simulink model "ActingHealthCheck"  (R2023a)
settings: Solver=VariableStepAuto  StartTime=0.0  StopTime=10.0  RelTol=1e-3
settings Model: Creator=aan18022  LastModifiedBy=aan18022

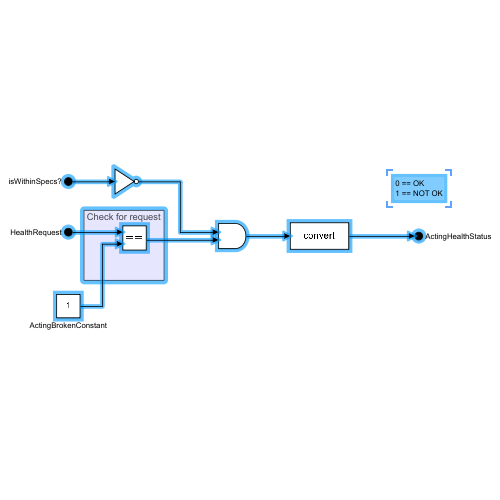
[thumbnail: Simulink's stored preview of the top-level diagram]
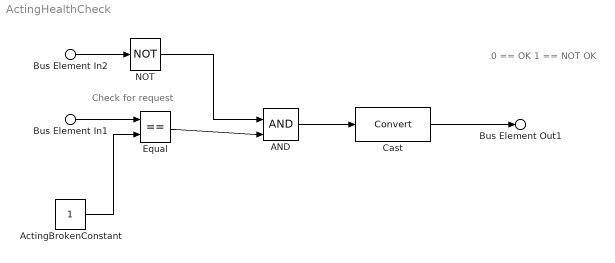
== system ActingHealthCheck ==
  note: 0 == OK
      | 1 == NOT OK
  note: Check for request
  Bus Element In1 : Inport  PortName=HealthRequest
  Bus Element In2 : Inport  Port=2  PortName=isWithinSpecs?
  AND : Logic  IconShape=distinctive  AllPortsSameDT=off  OutDataTypeStr=boolean
  ActingBrokenConstant : Constant
  Cast : DataTypeConversion  SaturateOnIntegerOverflow=off  RndMeth=Floor
  Equal : RelationalOperator  Operator===  OutDataTypeStr=boolean  RndMeth=Simplest  InputSameDT=off
  NOT : Logic  Operator=NOT  IconShape=distinctive  AllPortsSameDT=off  OutDataTypeStr=boolean
  Bus Element Out1 : Outport  PortName=ActingHealthStatus
  wires:
  Bus Element In1/1 -> Equal/1
  AND/1 -> Cast/1
  Bus Element In2/1 -> NOT/1
  Equal/1 -> AND/2
  Cast/1 -> Bus Element Out1/1
  NOT/1 -> AND/1
  ActingBrokenConstant/1 -> Equal/2
